simulink model "view_mech_explorer"  (R2023b)
settings: Solver=VariableStepAuto  StartTime=0.0  StopTime=1  RelTol=1e-3
model workspace (MAT data in the model file):
  pendulum_type = Simulink.Parameter
  pendulum_type.Value = 1
  pendulum_type.DataType = 'uint8'
  pendulum_type.DocUnits = '1'
  pendulum_type.Complexity = 'real'
  pendulum_type.Dimensions = [1 1]
undefined symbols (not defined in the file): pendulum_mass, Ts
libraries: fl_lib x2, nesl_utility x1
settings Model: DataDictionary=data_interface.sldd  Creator=upattacini  LastModifiedBy=upattacini
settings DataIOCC: SaveOutput=off  SignalLogging=off  DSMLogging=off  SaveTime=off  ReturnWorkspaceOutputs=off
settings ExplorerConfigSet: InternalSimMechanicsExplorerSettings="<ExplorerConfiguration><canonicalview>default</canonicalview><AnimationSetting><BasePlaybackSpeed>1.0</BasePlaybackSpeed><PlaybackSpeedFactor>1.0</PlaybackSpeedFactor></AnimationSetting><TilePanel><TileInfo><Tiles Columns=\"1\" Count=\"1\" Rows=\"1\"><Column Weight=\"1\"/><Row Weight=\"1\"/><Tile Height=\"1\" Width=\"1\" X=\"0\" Y=\"0\"/></Tiles></TileInfo><SceneInfo><SceneViewer><BGColor><R>0.60000002384185791</R><G>0.60000002384185791</G><B>0.60000002384185791</B></BGColor><Camera><DoPerspective>off</DoPerspective><Position><X>0.0138410343925078685</X><Y>-0.282265129449846885</Y><Z>1.00000000000000022</Z></Position><Center><X>0.0138410343925078685</X><Y>-0.282265129449846885</Y><Z>2.22044604925031308e-16</Z></Center><Up><X>0</X><Y>1</Y><Z>-0</Z></Up><ViewLimDist>1</ViewLimDist><YLim>0.631458368488044708</YLim><XLim>0.844014048337693001</XLim></Camera></SceneViewer></SceneInfo></TilePanel><MechEditorPanel><Cameras/><GfxPanelCameraMap/><VideoCreator><PlaybackSpeedRatio>1.0</PlaybackSpeedRatio><FrameRate>30</FrameRate><VideoFormat>Motion JPEG AVI</VideoFormat><FrameSize>auto</FrameSize></VideoCreator></MechEditorPanel></ExplorerConfiguration>"

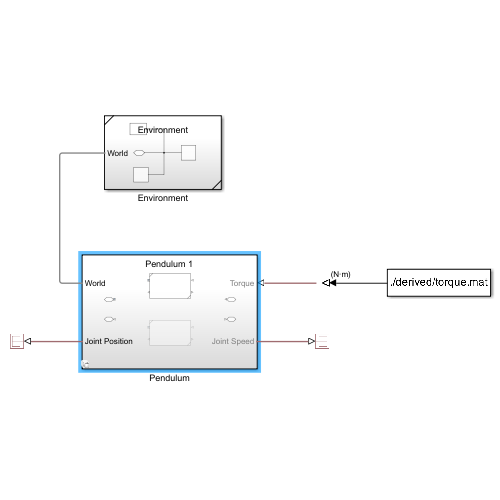
[thumbnail: Simulink's stored preview of the top-level diagram]
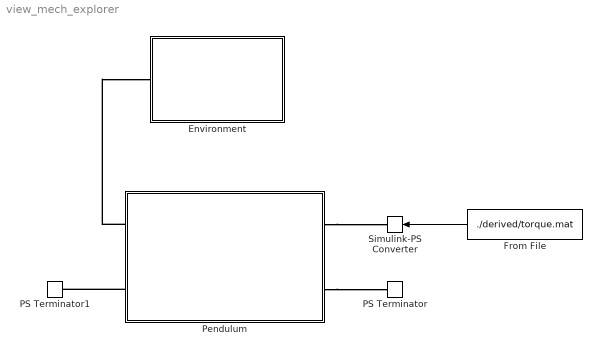
== system view_mech_explorer ==
  Environment : Subsystem  ReferencedSubsystem=Environment
      settings: PermitHierarchicalResolution=None
  From File : FromFile  FileName=./derived/torque.mat  SampleTime=Ts  ExtrapolationBeforeFirstDataPoint=Hold first value  InterpolationWithinTimeRange=Zero order hold  ExtrapolationAfterLastDataPoint=Hold last value
  PS Terminator : fl_lib/Physical Signals/Sinks/PS Terminator
  PS Terminator1 : fl_lib/Physical Signals/Sinks/PS Terminator
  Pendulum : Subsystem  Variant=on  VariantControl=Pendulum
  Simulink-PS Converter : nesl_utility/Simulink-PS Converter  PhysicalDomain=network_engine_domain  SubClassName=ps_input  LeftPortType=input  RightPortType=output  PseudoPeriodic=off  Frequencies=[]  NoiseDistribution=none  NoiseParameters=[]  Unit=N*m  AffineConversion=off  FilteringAndDerivatives=provide  SimscapeFilterOrder=1  InputFilterTimeConstant=0.001  UdotUserProvided=0
  wires:
  From File/1 -> Simulink-PS Converter/1
  connections:
  Pendulum/LConn1 -- Environment/LConn1
  Pendulum/LConn2 -- PS Terminator1/LConn1
  Pendulum/RConn1 -- Simulink-PS Converter/RConn1
  Pendulum/RConn2 -- PS Terminator/LConn1

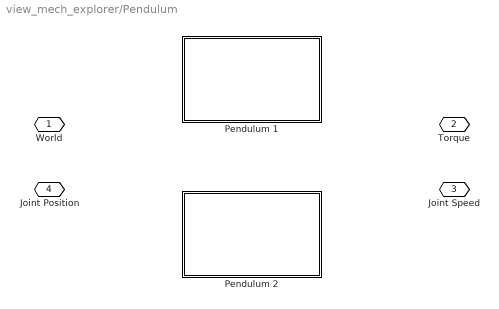
== system view_mech_explorer/Pendulum ==
  Pendulum 1 : Subsystem  VariantControl=pendulum_type == 1  ReferencedSubsystem=Pendulum  l=pendulum_1_length  m=pendulum_mass
      settings: PermitHierarchicalResolution=None
  Pendulum 2 : Subsystem  VariantControl=pendulum_type == 2  ReferencedSubsystem=Pendulum  l=pendulum_2_length  m=pendulum_mass
      settings: PermitHierarchicalResolution=None
  World : PMIOPort  Side=Left
  Torque : PMIOPort  Port=2  Side=Right
  Joint Speed : PMIOPort  Port=3  Side=Right
  Joint Position : PMIOPort  Port=4  Side=Left
